simulink model "sim_model_ver_tp2_V2_18a"  (R2018a)
settings: Solver=FixedStepAuto  StartTime=0.0  StopTime=150  FixedStep=0.01  RelTol=1e-3
libraries: simulink x3, powerlib_meascontrol x1
settings Model: Creator=eduhamel01  LastModifiedBy=zeiph

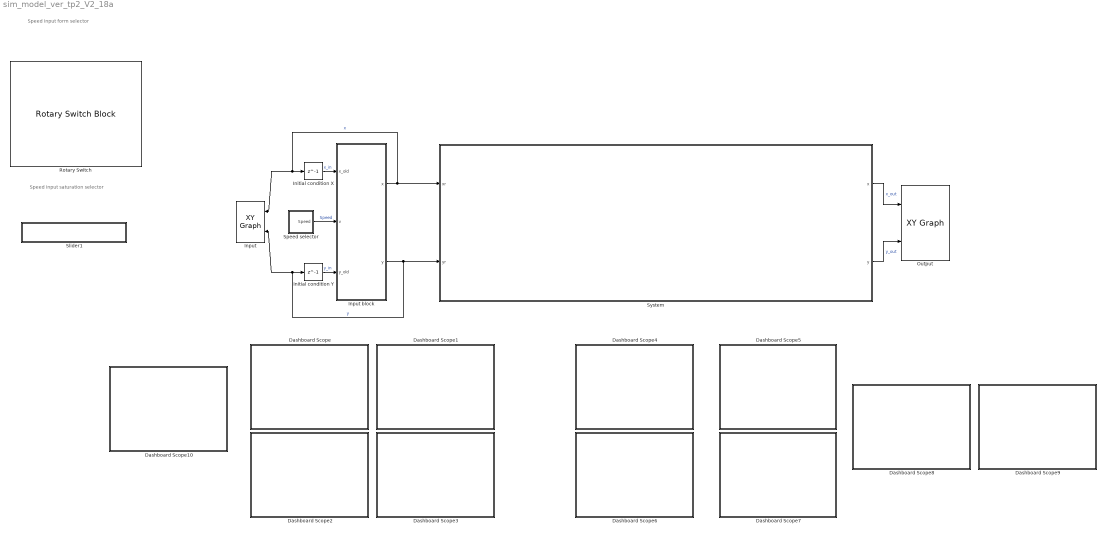
== system sim_model_ver_tp2_V2_18a ==
  note: Speed input form selector
  note: Speed input saturation
      | selector
  Dashboard Scope : Subsystem  DialogController=hmiCreateDDGDialog  IsWebBlock=on  mask(MWDashboardBlock){webBlockId=c4de3715-9afb-4af1-a433-5170b52d3f28, webBlockType=sdiscope, ShowInLibBrowser=on, ShowInitialText=on, HMISrcModelName=sim_model_ver_tp2_V2_18a}
      mask prompts: webBlockId "WebBlock Id"; webBlockType "WebBlock Type"; HMISrcModelName "Source Model"
      mask help: Traces signals on the dashboard scope during simulation.
      mask Help: helpview([docroot '/mapfiles/simulink.map'], 'hmi_scope')
      mask Display:
      | if strcmp(get_param(bdroot(gcb),'BlockDiagramType'),'library')
      |  image([(matlabroot) '/toolbox/simulink/hmi/icons/SDIScope.png'])
      | end
  Dashboard Scope1 : Subsystem  DialogController=hmiCreateDDGDialog  IsWebBlock=on  mask(MWDashboardBlock){webBlockId=d8a0ea41-111a-4039-b9d1-f6507a0fa386, webBlockType=sdiscope, ShowInLibBrowser=on, ShowInitialText=on, HMISrcModelName=sim_model_ver_tp2_V2_18a}
      mask prompts: webBlockId "WebBlock Id"; webBlockType "WebBlock Type"; HMISrcModelName "Source Model"
      mask help: Traces signals on the dashboard scope during simulation.
      mask Help: helpview([docroot '/mapfiles/simulink.map'], 'hmi_scope')
      mask Display:
      | if strcmp(get_param(bdroot(gcb),'BlockDiagramType'),'library')
      |  image([(matlabroot) '/toolbox/simulink/hmi/icons/SDIScope.png'])
      | end
  Dashboard Scope10 : Subsystem  DialogController=hmiCreateDDGDialog  IsWebBlock=on  mask(MWDashboardBlock){webBlockId=e598c93b-2c30-46a0-bf0d-6fba925e7910, webBlockType=sdiscope, ShowInLibBrowser=on, ShowInitialText=on, HMISrcModelName=sim_model_ver_tp2_V2_18a}
      mask prompts: webBlockId "WebBlock Id"; webBlockType "WebBlock Type"; HMISrcModelName "Source Model"
      mask help: Traces signals on the dashboard scope during simulation.
      mask Help: helpview([docroot '/mapfiles/simulink.map'], 'hmi_scope')
      mask Display:
      | if strcmp(get_param(bdroot(gcb),'BlockDiagramType'),'library')
      |  image([(matlabroot) '/toolbox/simulink/hmi/icons/SDIScope.png'])
      | end
  Dashboard Scope2 : Subsystem  DialogController=hmiCreateDDGDialog  IsWebBlock=on  mask(MWDashboardBlock){webBlockId=4159cd57-e175-4fa1-a47d-f6cec6e1deea, webBlockType=sdiscope, ShowInLibBrowser=on, ShowInitialText=on, HMISrcModelName=sim_model_ver_tp2_V2_18a}
      mask prompts: webBlockId "WebBlock Id"; webBlockType "WebBlock Type"; HMISrcModelName "Source Model"
      mask help: Traces signals on the dashboard scope during simulation.
      mask Help: helpview([docroot '/mapfiles/simulink.map'], 'hmi_scope')
      mask Display:
      | if strcmp(get_param(bdroot(gcb),'BlockDiagramType'),'library')
      |  image([(matlabroot) '/toolbox/simulink/hmi/icons/SDIScope.png'])
      | end
  Dashboard Scope3 : Subsystem  DialogController=hmiCreateDDGDialog  IsWebBlock=on  mask(MWDashboardBlock){webBlockId=daef7da9-74b8-43c7-82fc-7795073fa11e, webBlockType=sdiscope, ShowInLibBrowser=on, ShowInitialText=on, HMISrcModelName=sim_model_ver_tp2_V2_18a}
      mask prompts: webBlockId "WebBlock Id"; webBlockType "WebBlock Type"; HMISrcModelName "Source Model"
      mask help: Traces signals on the dashboard scope during simulation.
      mask Help: helpview([docroot '/mapfiles/simulink.map'], 'hmi_scope')
      mask Display:
      | if strcmp(get_param(bdroot(gcb),'BlockDiagramType'),'library')
      |  image([(matlabroot) '/toolbox/simulink/hmi/icons/SDIScope.png'])
      | end
  Dashboard Scope4 : Subsystem  DialogController=hmiCreateDDGDialog  IsWebBlock=on  mask(MWDashboardBlock){webBlockId=15f50f5f-b6af-4a54-ad88-f1adc314ec68, webBlockType=sdiscope, ShowInLibBrowser=on, ShowInitialText=on, HMISrcModelName=sim_model_ver_tp2_V2_18a}
      mask prompts: webBlockId "WebBlock Id"; webBlockType "WebBlock Type"; HMISrcModelName "Source Model"
      mask help: Traces signals on the dashboard scope during simulation.
      mask Help: helpview([docroot '/mapfiles/simulink.map'], 'hmi_scope')
      mask Display:
      | if strcmp(get_param(bdroot(gcb),'BlockDiagramType'),'library')
      |  image([(matlabroot) '/toolbox/simulink/hmi/icons/SDIScope.png'])
      | end
  Dashboard Scope5 : Subsystem  DialogController=hmiCreateDDGDialog  IsWebBlock=on  mask(MWDashboardBlock){webBlockId=ec3d15d5-e346-476a-ad8c-d1b086a68142, webBlockType=sdiscope, ShowInLibBrowser=on, ShowInitialText=on, HMISrcModelName=sim_model_ver_tp2_V2_18a}
      mask prompts: webBlockId "WebBlock Id"; webBlockType "WebBlock Type"; HMISrcModelName "Source Model"
      mask help: Traces signals on the dashboard scope during simulation.
      mask Help: helpview([docroot '/mapfiles/simulink.map'], 'hmi_scope')
      mask Display:
      | if strcmp(get_param(bdroot(gcb),'BlockDiagramType'),'library')
      |  image([(matlabroot) '/toolbox/simulink/hmi/icons/SDIScope.png'])
      | end
  Dashboard Scope6 : Subsystem  DialogController=hmiCreateDDGDialog  IsWebBlock=on  mask(MWDashboardBlock){webBlockId=ade469b5-ab36-48eb-aed8-0e4712d40a23, webBlockType=sdiscope, ShowInLibBrowser=on, ShowInitialText=on, HMISrcModelName=sim_model_ver_tp2_V2_18a}
      mask prompts: webBlockId "WebBlock Id"; webBlockType "WebBlock Type"; HMISrcModelName "Source Model"
      mask help: Traces signals on the dashboard scope during simulation.
      mask Help: helpview([docroot '/mapfiles/simulink.map'], 'hmi_scope')
      mask Display:
      | if strcmp(get_param(bdroot(gcb),'BlockDiagramType'),'library')
      |  image([(matlabroot) '/toolbox/simulink/hmi/icons/SDIScope.png'])
      | end
  Dashboard Scope7 : Subsystem  DialogController=hmiCreateDDGDialog  IsWebBlock=on  mask(MWDashboardBlock){webBlockId=6b8597d2-3432-4ff4-afe4-566152607966, webBlockType=sdiscope, ShowInLibBrowser=on, ShowInitialText=on, HMISrcModelName=sim_model_ver_tp2_V2_18a}
      mask prompts: webBlockId "WebBlock Id"; webBlockType "WebBlock Type"; HMISrcModelName "Source Model"
      mask help: Traces signals on the dashboard scope during simulation.
      mask Help: helpview([docroot '/mapfiles/simulink.map'], 'hmi_scope')
      mask Display:
      | if strcmp(get_param(bdroot(gcb),'BlockDiagramType'),'library')
      |  image([(matlabroot) '/toolbox/simulink/hmi/icons/SDIScope.png'])
      | end
  Dashboard Scope8 : Subsystem  DialogController=hmiCreateDDGDialog  IsWebBlock=on  mask(MWDashboardBlock){webBlockId=943eea54-2769-4f1e-b72b-d64844e3b961, webBlockType=sdiscope, ShowInLibBrowser=on, ShowInitialText=on, HMISrcModelName=sim_model_ver_tp2_V2_18a}
      mask prompts: webBlockId "WebBlock Id"; webBlockType "WebBlock Type"; HMISrcModelName "Source Model"
      mask help: Traces signals on the dashboard scope during simulation.
      mask Help: helpview([docroot '/mapfiles/simulink.map'], 'hmi_scope')
      mask Display:
      | if strcmp(get_param(bdroot(gcb),'BlockDiagramType'),'library')
      |  image([(matlabroot) '/toolbox/simulink/hmi/icons/SDIScope.png'])
      | end
  Dashboard Scope9 : Subsystem  DialogController=hmiCreateDDGDialog  IsWebBlock=on  mask(MWDashboardBlock){webBlockId=c38c5079-8b06-4ba5-8b65-f880e239962a, webBlockType=sdiscope, ShowInLibBrowser=on, ShowInitialText=on, HMISrcModelName=sim_model_ver_tp2_V2_18a}
      mask prompts: webBlockId "WebBlock Id"; webBlockType "WebBlock Type"; HMISrcModelName "Source Model"
      mask help: Traces signals on the dashboard scope during simulation.
      mask Help: helpview([docroot '/mapfiles/simulink.map'], 'hmi_scope')
      mask Display:
      | if strcmp(get_param(bdroot(gcb),'BlockDiagramType'),'library')
      |  image([(matlabroot) '/toolbox/simulink/hmi/icons/SDIScope.png'])
      | end
  Initial condition X : Delay  DelayLength=1
  Initial condition Y : Delay  DelayLength=1
  Input : simulink/Sinks/XY Graph  xmin=-1  xmax=5.5  ymin=-5  ymax=20  st=-1
  Input block : MATLAB Function  TreatAsAtomicUnit=on
  Output : simulink/Sinks/XY Graph  xmin=-1  xmax=5.5  ymin=-5  ymax=20  st=-1
  Rotary Switch : RotarySwitchBlock  WebBlockId=188
      settings: Values={{'Constant', 'Sine', 'Pulse', 'Ramp', 'Triangle'}, [1 2 3 4 5]}
  Slider1 : Subsystem  DialogController=hmiCreateDDGDialog  IsWebBlock=on  mask(MWDashboardBlock){webBlockId=67a2eff1-47b2-4bb7-ad0b-84707d92850e, webBlockType=slider, ShowInLibBrowser=on, ShowInitialText=on, HMISrcModelName=sim_model_ver_tp2_V2_18a}
      mask prompts: webBlockId "WebBlock Id"; webBlockType "WebBlock Type"; HMISrcModelName "Source Model"
      mask help: Set value to tune parameters or variables.
      mask Help: helpview([docroot '/mapfiles/simulink.map'], 'hmi_slider')
      mask Display:
      | if strcmp(get_param(bdroot(gcb),'BlockDiagramType'),'library')
      |  image([(matlabroot) '/toolbox/simulink/hmi/icons/Slider.png'])
      | end
  Speed selector : Subsystem
  System : Subsystem
  wires:
  System/1(x) -> Output/1  "x_out"
  System/2(y) -> Output/2  "y_out"
  Initial condition X/1 -> Input block/1(x_old)  "x_in"
  Input block/1(x) -> Initial condition X/1, Input/1, System/1(xr)  "x"
  Initial condition Y/1 -> Input block/3(y_old)  "y_in"
  Input block/2(y) -> Input/2, Initial condition Y/1, System/2(yr)  "y"
  Speed selector/1(Speed) -> Input block/2(v)  "Speed"

== system sim_model_ver_tp2_V2_18a/Dashboard Scope ==

== system sim_model_ver_tp2_V2_18a/Dashboard Scope1 ==

== system sim_model_ver_tp2_V2_18a/Dashboard Scope10 ==

== system sim_model_ver_tp2_V2_18a/Dashboard Scope2 ==

== system sim_model_ver_tp2_V2_18a/Dashboard Scope3 ==

== system sim_model_ver_tp2_V2_18a/Dashboard Scope4 ==

== system sim_model_ver_tp2_V2_18a/Dashboard Scope5 ==

== system sim_model_ver_tp2_V2_18a/Dashboard Scope6 ==

== system sim_model_ver_tp2_V2_18a/Dashboard Scope7 ==

== system sim_model_ver_tp2_V2_18a/Dashboard Scope8 ==

== system sim_model_ver_tp2_V2_18a/Dashboard Scope9 ==

== system sim_model_ver_tp2_V2_18a/Slider1 ==

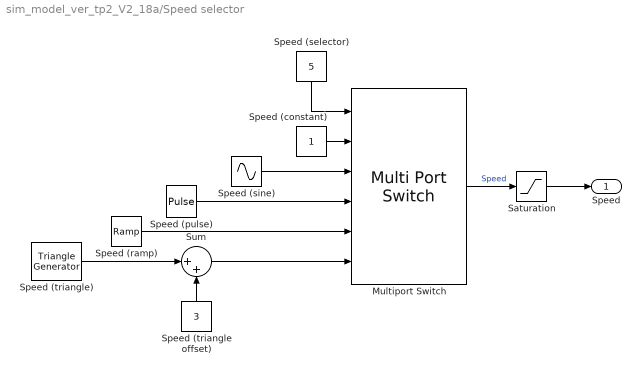
== system sim_model_ver_tp2_V2_18a/Speed selector ==
  Multiport Switch : MultiPortSwitch  Inputs=5
  Saturation : Saturate  UpperLimit=4.664899955035971
  Speed (constant) : Constant
  Speed (pulse) : DiscretePulseGenerator  PulseType=Time based  Period=10  PulseWidth=50
  Speed (ramp) : simulink/Sources/Ramp  slope=1  start=0  InitialOutput=0
  Speed (selector) : Constant  Value=5
  Speed (sine) : Sin  Bias=1  SampleTime=0
  Speed (triangle offset) : Constant  Value=3
  Speed (triangle) : powerlib_meascontrol/Pulse & Signal Generators/Triangle Generator  Freq=1/30  Phase=90  Ts=0
  Sum : Sum  Inputs=|++
  Speed : Outport
  wires:
  Speed (triangle offset)/1 -> Sum/2
  Sum/1 -> Multiport Switch/6
  Speed (pulse)/1 -> Multiport Switch/4
  Speed (triangle)/1 -> Sum/1
  Speed (sine)/1 -> Multiport Switch/3
  Speed (constant)/1 -> Multiport Switch/2
  Speed (selector)/1 -> Multiport Switch/1
  Speed (ramp)/1 -> Multiport Switch/5
  Multiport Switch/1 -> Saturation/1  "Speed"
  Saturation/1 -> Speed/1

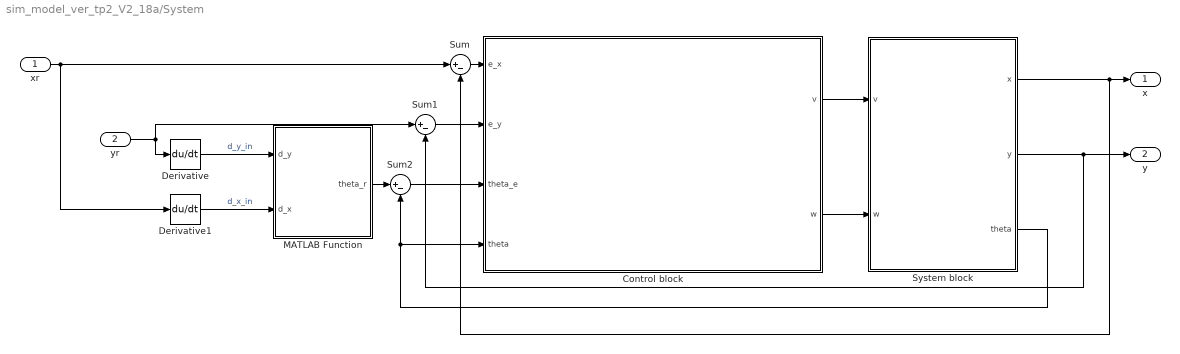
== system sim_model_ver_tp2_V2_18a/System ==
  xr : Inport
  yr : Inport  Port=2
  Control block : Subsystem
  Derivative : Derivative
  Derivative1 : Derivative
  MATLAB Function : MATLAB Function  TreatAsAtomicUnit=on
  Sum : Sum  Inputs=|+-
  Sum1 : Sum  Inputs=|+-
  Sum2 : Sum  Inputs=|+-
  System block : Subsystem
  x : Outport  VectorParamsAs1DForOutWhenUnconnected=off
  y : Outport  Port=2  VectorParamsAs1DForOutWhenUnconnected=off
  wires:
  Sum1/1 -> Control block/2(e_y)
  Control block/2(w) -> System block/2(w)
  Derivative/1 -> MATLAB Function/1(d_y)  "d_y_in"
  MATLAB Function/1(theta_r) -> Sum2/1
  System block/2(y) -> y/1, Sum1/2
  System block/3(theta) -> Control block/4(theta), Sum2/2
  System block/1(x) -> x/1, Sum/2
  Derivative1/1 -> MATLAB Function/2(d_x)  "d_x_in"
  Sum/1 -> Control block/1(e_x)
  Control block/1(v) -> System block/1(v)
  Sum2/1 -> Control block/3(theta_e)
  yr/1 -> Derivative/1, Sum1/1
  xr/1 -> Sum/1, Derivative1/1

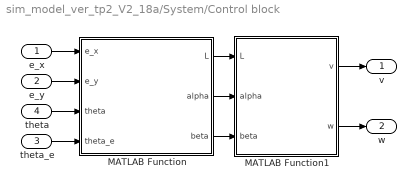
== system sim_model_ver_tp2_V2_18a/System/Control block ==
  e_x : Inport
  e_y : Inport  Port=2
  theta_e : Inport  Port=3
  theta : Inport  Port=4
  MATLAB Function : MATLAB Function  TreatAsAtomicUnit=on
  MATLAB Function1 : MATLAB Function  TreatAsAtomicUnit=on
  v : Outport  VectorParamsAs1DForOutWhenUnconnected=off
  w : Outport  Port=2  VectorParamsAs1DForOutWhenUnconnected=off
  wires:
  MATLAB Function1/1(v) -> v/1
  MATLAB Function1/2(w) -> w/1
  e_x/1 -> MATLAB Function/1(e_x)
  e_y/1 -> MATLAB Function/2(e_y)
  theta_e/1 -> MATLAB Function/4(theta_e)
  MATLAB Function/1(L) -> MATLAB Function1/1(L)
  MATLAB Function/2(alpha) -> MATLAB Function1/2(alpha)
  MATLAB Function/3(beta) -> MATLAB Function1/3(beta)
  theta/1 -> MATLAB Function/3(theta)

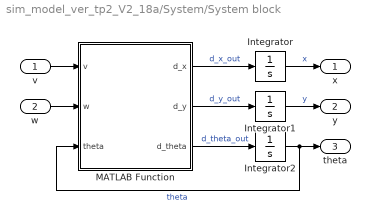
== system sim_model_ver_tp2_V2_18a/System/System block ==
  v : Inport
  w : Inport  Port=2
  Integrator : Integrator
  Integrator1 : Integrator
  Integrator2 : Integrator
  MATLAB Function : MATLAB Function  TreatAsAtomicUnit=on
  x : Outport  VectorParamsAs1DForOutWhenUnconnected=off
  y : Outport  Port=2  VectorParamsAs1DForOutWhenUnconnected=off
  theta : Outport  Port=3  VectorParamsAs1DForOutWhenUnconnected=off
  wires:
  Integrator2/1 -> theta/1, MATLAB Function/3(theta)  "theta"
  MATLAB Function/1(d_x) -> Integrator/1  "d_x_out"
  MATLAB Function/3(d_theta) -> Integrator2/1  "d_theta_out"
  v/1 -> MATLAB Function/1(v)
  MATLAB Function/2(d_y) -> Integrator1/1  "d_y_out"
  Integrator/1 -> x/1  "x"
  w/1 -> MATLAB Function/2(w)
  Integrator1/1 -> y/1  "y"

== matlab function sim_model_ver_tp2_V2_18a/System/Control block/MATLAB Function ==
  data: e_x input; L output; e_y input; theta input; theta_e input; alpha output; beta output
function [L , alpha, beta] = to_parameters(e_x , e_y , theta , theta_e)
    L = sqrt(e_x * e_x + e_y * e_y);
    alpha = mod(atan2(e_y , e_x) , 2*pi) - theta;
    beta = theta_e - alpha;
end

== matlab function sim_model_ver_tp2_V2_18a/System/System block/MATLAB Function ==
  data: v input; d_x output; w input; theta input; d_y output; d_theta output
function [d_x,  d_y,  d_theta] = system(v , w , theta)

    d_x = v*cos(theta);
    d_y = v*sin(theta);
    d_theta = w;

end

== matlab function sim_model_ver_tp2_V2_18a/System/Control block/MATLAB Function1 ==
  data: L input; v output; w output; alpha input; beta input
function [v , w] = to_v_w(L, alpha , beta)

%old
% k_L = -3;
% k_alpha = -210;
% k_beta = 4.5;


k_L = -5.5;
k_alpha = -220;
k_beta = 2;

v = -k_L * L;
w = -k_alpha * alpha - k_beta * beta;

end

== matlab function sim_model_ver_tp2_V2_18a/System/MATLAB Function ==
  data: d_y input; d_x input; theta_r output
function theta_r = arctan2(d_y , d_x)
    theta_r = mod(atan2(d_y , d_x) , 2*pi);
end

== matlab function sim_model_ver_tp2_V2_18a/Input block ==
  data: x output; x_old input; v input; y_old input; y output
function [x, y] = input(x_old , v , y_old)

    h = 10; %Straight line distance
    d = 5; %"Circle" diameter
    
    Ts = 0.01; %MUST also Simulink sample time

    is_on_part_1_flag = ((x_old == 0 && y_old < h));
    is_on_part_2_flag = ((x_old < d && y_old >= h));
    is_on_part_3_flag = ((x_old >= d && y_old >=0));
    is_on_part_4_flag = (~is_on_part_1_flag &&...
                         ~is_on_part_2_flag &&...
                         ~is_on_part_3_flag);
  
                     
         
    x = is_on_part_1_flag * (0)+...
        is_on_part_2_flag * (x_old + Ts*v)+... 
        is_on_part_3_flag * (d)+...
        is_on_part_4_flag * ((x_old - Ts*v > 0)*(x_old - Ts*v)); %Ternary operator workaround

    y = is_on_part_1_flag * (y_old + Ts*v)+...
        is_on_part_2_flag * (h + (d/2)*sin(pi*x/d))+... 
        is_on_part_3_flag * (y_old - Ts*v)+...
        is_on_part_4_flag * (- (d/2)*sin(pi*x/d));    

         
%     x = is_on_part_1_flag * (0)+...
%         is_on_part_2_flag * (timestamp*v)+... 
%         is_on_part_3_flag * (d)+...
%         is_on_part_4_flag * ((d - timestamp*v >0)*(d - timestamp*v));
%    
%     y = is_on_part_1_flag * (timestamp*v)+...
%         is_on_part_2_flag * (h + (d/2) * sin(pi*timestamp*v/d))+... 
%         is_on_part_3_flag * (h-timestamp*v)+...
%         is_on_part_4_flag * (-(d/2) * sin(pi*timestamp*v/d));
 

            
            


end
